simulink library "plantModel_cl"  (R2020a)
settings: Solver=VariableStepAuto  StartTime=0.0  StopTime=10.0  RelTol=1e-3
libraries: shared6dof x1, simulink x1, calcAeroForcesInB x1, calcTangentialCoord_ul x1, calcThrDrag_ul x1
settings Model: Creator=Ayaz  LastModifiedBy=Ayaz

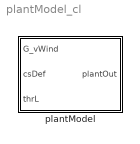
== system plantModel_cl ==
  plantModel : Subsystem  mask{kiteMass=36.8, kiteJmat=eye(3), refChord=0.55, refSpan=5.5, refArea=3, xme_0=[0 0 0], Vm_0=[0 0 0], eul_0=[0 0 0], pm_0=[0 0 0], dThr=0, CdThr=0, rhoAir=1.225, gravAccl=0}
      mask prompts: kiteMass "Kite mass [kg]"; kiteJmat "Kite inertia matrix [kg-m^2]"; refChord "Kite reference chord [m]"; refSpan "Kite reference span [m]"; refArea "Kite reference area [m^2]"; xme_0 "Initial position in the inertial frame [m]"; Vm_0 "Initial velocity in the body frame [m/s]"; eul_0 "Initial Euler angles [rad]"; pm_0 "Initial angular velocity [rad/s]"; dThr "Tether diameter [m]"; CdThr "Tether drag coefficient [-]"; rhoAir "Air density [kg/m^3]"; gravAccl "Gravitational acceleration [m/s^2]"
      mask TypeOptions kiteMass: 6DOF (Euler Angles)/mass_0
      mask TypeOptions kiteJmat: 6DOF (Euler Angles)/inertia
      mask TypeOptions refChord: calcAeroLoads/refChord
      mask TypeOptions refSpan: calcAeroLoads/refSpan
      mask TypeOptions refArea: calcAeroLoads/refArea
      mask TypeOptions xme_0: 6DOF (Euler Angles)/xme_0
      mask TypeOptions Vm_0: 6DOF (Euler Angles)/Vm_0
      mask TypeOptions eul_0: 6DOF (Euler Angles)/eul_0
      mask TypeOptions pm_0: 6DOF (Euler Angles)/pm_0
      mask TypeOptions dThr: tetherDrag/dThr
      mask TypeOptions CdThr: tetherDrag/CdThr
      mask TypeOptions rhoAir: calcAeroLoads/rhoAir | tetherDrag/rhoAir
      mask DialogControl ParameterGroupVar Prompt: Kite parameters
      mask DialogControl Container3 Prompt: Initial conditions
      mask DialogControl Container5 Prompt: Tether parameters
      mask DialogControl Container4 Prompt: Environment parameters

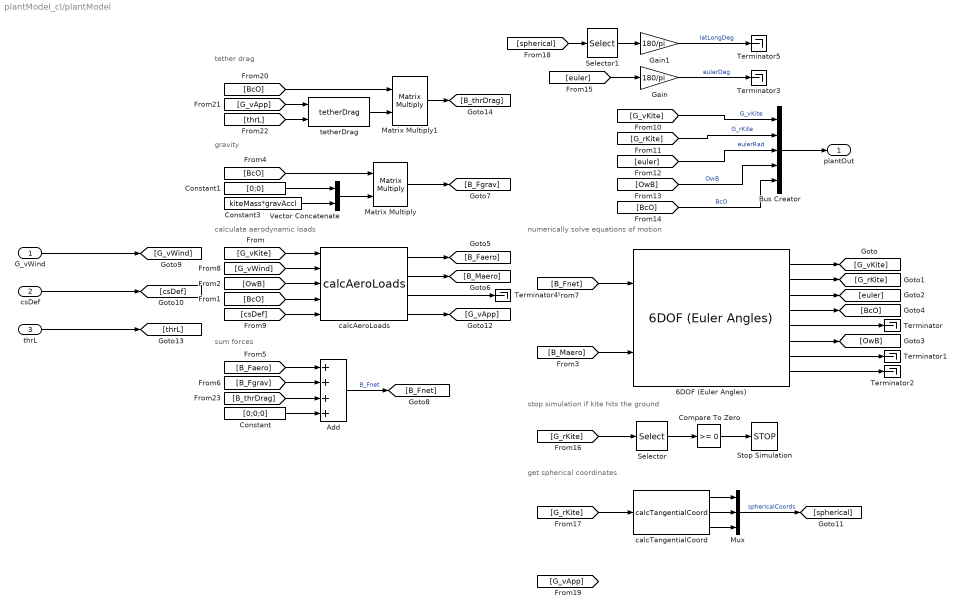
== system plantModel_cl/plantModel ==
  note: tether drag
  note: get spherical coordinates
  note: stop simulation if kite hits the ground
  note: calculate aerodynamic loads
  note: numerically solve equations of motion
  note: sum forces
  note: gravity
  G_vWind : Inport
  csDef : Inport  Port=2
  thrL : Inport  Port=3
  6DOF (Euler Angles) : shared6dof/6DOF (Euler Angles)  units=Metric (MKS)  mtype=Fixed  rep=Euler Angles  xme_0=xme_0  Vm_0=Vm_0  eul_0=eul_0  pm_0=pm_0  mass_0=kiteMass  mass_e=0.5  mass_f=2.0  inertia=kiteJmat  inertia_e=eye(3)  inertia_f=2*eye(3)  k_quat=1.0  vre_flag=on  abi_flag=off  aMode=0  xme_statename=''  Vm_statename=''  eul_statename=''  quat_statename=''  pm_statename=''  mass_statename=''
      settings: SourceProductBaseCode=AE,PW,MT,VE,VP
  Add : Sum  Inputs=++++
  Bus Creator : BusCreator  Inputs=5
  Compare To Zero : simulink/Logic and Bit Operations/Compare To Zero  relop=>=  OutDataTypeStr=boolean
  Constant : Constant  Value=[0;0;0]
  Constant1 : Constant  Value=[0;0]  VectorParams1D=off
  Constant3 : Constant  Value=kiteMass*gravAccl
  Gain : Gain  Gain=180/pi
  Gain1 : Gain  Gain=180/pi
  Matrix Multiply : Product  Multiplication=Matrix(*)
  Matrix Multiply1 : Product  Multiplication=Matrix(*)
  Mux : Mux  Inputs=3
  Selector : Selector  InputPortWidth=3  IndexOptions=Index vector (dialog)  Indices=3  OutputSizes=1
  Selector1 : Selector  InputPortWidth=3  IndexOptions=Index vector (dialog)  Indices=[1 2]  OutputSizes=1
  Stop Simulation : Stop
  Terminator{,1..5} (6 alike) : Terminator
  Vector Concatenate : Concatenate
  calcAeroLoads : calcAeroForcesInB/calcAeroLoads  refChord=refChord  refSpan=refSpan  refArea=refArea  rhoAir=rhoAir
  calcTangentialCoord : calcTangentialCoord_ul/calcTangentialCoord  SystemSampleTime=-1  Latency=0  AutoFrameSizeCalculation=off
  tetherDrag : calcThrDrag_ul/tetherDrag  dThr=dThr  CdThr=CdThr  rhoAir=rhoAir
  plantOut : Outport
  wires:
  6DOF (Euler Angles)/1 -> [G_vKite]
  [G_vKite] -> calcAeroLoads/1
  6DOF (Euler Angles)/2 -> [G_rKite]
  6DOF (Euler Angles)/3 -> [euler]
  6DOF (Euler Angles)/6 -> [OwB]
  6DOF (Euler Angles)/4 -> [BcO]
  [BcO] -> calcAeroLoads/4
  [OwB] -> calcAeroLoads/3
  calcAeroLoads/1 -> [B_Faero]
  calcAeroLoads/2 -> [B_Maero]
  [B_Maero] -> 6DOF (Euler Angles)/2
  Constant3/1 -> Vector Concatenate/2
  Constant1/1 -> Vector Concatenate/1
  Vector Concatenate/1 -> Matrix Multiply/2
  [BcO] -> Matrix Multiply/1
  Matrix Multiply/1 -> [B_Fgrav]
  [B_Faero] -> Add/1
  [B_Fgrav] -> Add/2
  Add/1 -> [B_Fnet]  "B_Fnet"
  [B_Fnet] -> 6DOF (Euler Angles)/1
  [G_vWind] -> calcAeroLoads/2
  [csDef] -> calcAeroLoads/5
  G_vWind/1 -> [G_vWind]
  [G_vKite] -> Bus Creator/1  "G_vKite"
  [G_rKite] -> Bus Creator/2  "G_rKite"
  [euler] -> Bus Creator/3  "eulerRad"
  [OwB] -> Bus Creator/4  "OwB"
  Bus Creator/1 -> plantOut/1
  [BcO] -> Bus Creator/5  "BcO"
  6DOF (Euler Angles)/5 -> Terminator/1
  6DOF (Euler Angles)/7 -> Terminator1/1
  6DOF (Euler Angles)/8 -> Terminator2/1
  csDef/1 -> [csDef]
  [euler] -> Gain/1
  Gain/1 -> Terminator3/1  "eulerDeg"
  [G_rKite] -> Selector/1
  Selector/1 -> Compare To Zero/1
  Compare To Zero/1 -> Stop Simulation/1
  [G_rKite] -> calcTangentialCoord/1
  Mux/1 -> [spherical]  "sphericalCoords"
  [spherical] -> Selector1/1
  Gain1/1 -> Terminator5/1  "latLongDeg"
  calcTangentialCoord/1 -> Mux/1
  calcTangentialCoord/2 -> Mux/2
  calcTangentialCoord/3 -> Mux/3
  Selector1/1 -> Gain1/1
  calcAeroLoads/4 -> [G_vApp]
  calcAeroLoads/3 -> Terminator4/1
  tetherDrag/1 -> Matrix Multiply1/2
  [BcO] -> Matrix Multiply1/1
  [G_vApp] -> tetherDrag/1
  thrL/1 -> [thrL]
  [thrL] -> tetherDrag/2
  Matrix Multiply1/1 -> [B_thrDrag]
  Constant/1 -> Add/4
  [B_thrDrag] -> Add/3
